simulink model "MMC_singlephase_test"  (Simulink 9.0)
settings: Solver=ode5  StartTime=0.0  StopTime=2  MaxStep=1e-4  RelTol=1e-3
libraries: powerlib x43
settings Model: Creator=lenovo  LastModifiedBy=lenovo
settings DataIOCC: SaveFormat=Dataset
settings OptimizationCC: LifeSpan=auto
settings DebuggingCC: UnderspecifiedInitializationDetection=Simplified  MergeDetectMultiDrivingBlocksExec=error  SFUnexpectedBacktrackingDiag=error  SFNoUnconditionalDefaultTransitionDiag=error  SFExecutionAtInitializationDiag=warning
settings HardwareCC: ProdBitPerPointer=64  ProdBitPerSizeT=64  ProdBitPerPtrDiffT=64  ProdLargestAtomicFloat=Float  ProdIntDivRoundTo=Zero  ProdEndianess=LittleEndian  ProdWordSize=64  ProdHWDeviceType=Intel->x86-64 (Windows64)
settings ModelReferenceCC: PropagateSignalLabelsOutOfModel=on
settings CodeAppCC: StateflowObjectComments=off
settings GRTTargetCC: TargetLangStandard=C99 (ISO)
settings ConfigComp: CovMetricSettings=dwe  CovHtmlReporting=off  CovSaveCumulativeToWorkspaceVar=off  CovSaveSingleToWorkspaceVar=off  CovExternalEMLEnable=on

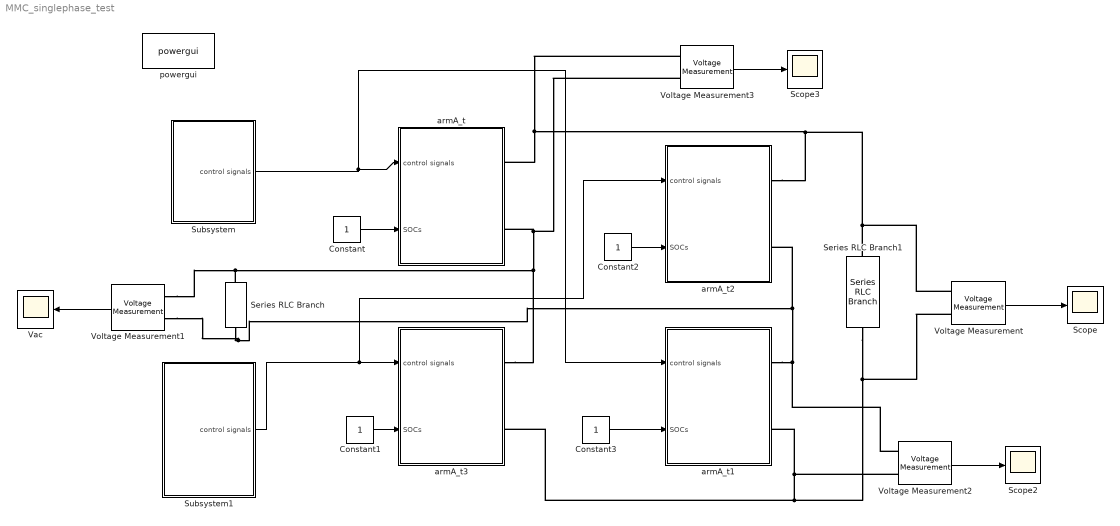
== system MMC_singlephase_test ==
  Constant{,1..3} (4 alike) : Constant
  Scope : Scope
  Scope2 : Scope
  Scope3 : Scope
  Series RLC Branch : powerlib/Elements/Series RLC Branch  LConnTagsString=__new0  RConnTagsString=__new0  BranchType=R  Resistance=1  Inductance=1e-3  SetiL0=off  InitialCurrent=0  Capacitance=1e-6  Setx0=off  InitialVoltage=0  Measurements=None
  Series RLC Branch1 : powerlib/Elements/Series RLC Branch  LConnTagsString=__new0  RConnTagsString=__new0  BranchType=R  Resistance=1  Inductance=1e-3  SetiL0=off  InitialCurrent=0  Capacitance=1e-6  Setx0=off  InitialVoltage=0  Measurements=None
  Subsystem : Subsystem
  Subsystem1 : Subsystem
  Vac : Scope
  Voltage Measurement{,1..3} (4 alike) : powerlib/Measurements/Voltage Measurement  PhasorSimulation=off  OutputType=Complex  PSBequivalent=0
  armA_t : Subsystem
  armA_t1 : Subsystem
  armA_t2 : Subsystem
  armA_t3 : Subsystem
  powergui : powerlib/powergui  Priority=1  SimulationMode=Discrete  SampleTime=50e-6  frequency=60  Iterations=50  frequencyindice=0  Pbase=100e6  ErrMax=1e-4  UnitsV=kV  UnitsW=MW  buscounter=0  FunctionMessages=off  echomessages=off  EnableUseOfTLC=off  CurrentSourceSwitches=off  DisableSnubberDevices=off  DisableRonSwitches=off  DisableVfSwitches=off  DisplayEquations=off  SolverType=Tustin/Backward Euler (TBE)  Interpol=off  ExternalGateDelay=off  methode=off  Ts=100  x0status=blocks  SPID=on  SwTol=0  HookPort=off  RestoreLinks=warning  ResistiveCurrentMeasurement=off  Frange=[0:2:500]  Ylog=off  Xlog=on  ShowGrid=off  save=off  variable=ZData  structure=0  ZoomFFT=off  StartTime=0.0  cycles=1  DisplayStyle=1  fundamental=60  FreqAxis=off  MaxFrequency=1000  frequencyindicesteady=1  RmsSteady=1  display=off
  wires:
  Voltage Measurement/1 -> Scope/1
  Subsystem/1(control signals) -> armA_t1/1(control signals), armA_t/1(control signals)
  Constant1/1 -> armA_t3/2(SOCs)
  Constant3/1 -> armA_t1/2(SOCs)
  Constant2/1 -> armA_t2/2(SOCs)
  Subsystem1/1(control signals) -> armA_t2/1(control signals), armA_t3/1(control signals)
  Voltage Measurement1/1 -> Vac/1
  Voltage Measurement2/1 -> Scope2/1
  Voltage Measurement3/1 -> Scope3/1
  Constant/1 -> armA_t/2(SOCs)
  connections:
  Series RLC Branch1/LConn1 -- Voltage Measurement/LConn1 -- armA_t/RConn1 -- Voltage Measurement3/LConn1 -- armA_t2/RConn1
  Series RLC Branch/LConn1 -- armA_t3/RConn1 -- armA_t/RConn2 -- Voltage Measurement3/LConn2 -- Voltage Measurement1/LConn1
  armA_t3/RConn2 -- Voltage Measurement/LConn2 -- Series RLC Branch1/RConn1 -- Voltage Measurement2/LConn2 -- armA_t1/RConn2
  Voltage Measurement1/LConn2 -- Series RLC Branch/RConn1 -- armA_t2/RConn2 -- armA_t1/RConn1 -- Voltage Measurement2/LConn1

== system MMC_singlephase_test/Subsystem ==
  Bus Creator : BusCreator  Inputs=3
  submodule1 : DiscretePulseGenerator  PulseType=Time based  Period=1  PulseWidth=75  PhaseDelay=0.125
  submodule2 : DiscretePulseGenerator  PulseType=Time based  Period=1  PulseWidth=50  PhaseDelay=0.25
  submodule3 : DiscretePulseGenerator  PulseType=Time based  Period=1  PulseWidth=25  PhaseDelay=0.375
  control signals : Outport
  wires:
  Bus Creator/1 -> control signals/1
  submodule1/1 -> Bus Creator/1
  submodule2/1 -> Bus Creator/2
  submodule3/1 -> Bus Creator/3

== system MMC_singlephase_test/Subsystem1 ==
  Bus Creator : BusCreator  Inputs=3
  Logical Operator : Logic  Operator=NOT  AllPortsSameDT=off  OutDataTypeStr=boolean
  Logical Operator1 : Logic  Operator=NOT  AllPortsSameDT=off  OutDataTypeStr=boolean
  Logical Operator2 : Logic  Operator=NOT  AllPortsSameDT=off  OutDataTypeStr=boolean
  submodule1 : DiscretePulseGenerator  PulseType=Time based  Period=1  PulseWidth=75  PhaseDelay=0.125
  submodule2 : DiscretePulseGenerator  PulseType=Time based  Period=1  PulseWidth=50  PhaseDelay=0.25
  submodule3 : DiscretePulseGenerator  PulseType=Time based  Period=1  PulseWidth=25  PhaseDelay=0.375
  control signals : Outport
  wires:
  Bus Creator/1 -> control signals/1
  submodule1/1 -> Logical Operator/1
  submodule2/1 -> Logical Operator1/1
  submodule3/1 -> Logical Operator2/1
  Logical Operator/1 -> Bus Creator/1
  Logical Operator1/1 -> Bus Creator/2
  Logical Operator2/1 -> Bus Creator/3

== system MMC_singlephase_test/armA_t ==
  control signals : Inport
  SOCs : Inport  Port=2
  Bus Selector : BusSelector  OutputSignals=signal1,signal2,signal3
  SubModule1 : Subsystem
  SubModule2 : Subsystem
  SubModule3 : Subsystem
  Conn1 : PMIOPort  Port=1  Side=Right
  Conn2 : PMIOPort  Port=2  Side=Right
  wires:
  control signals/1 -> Bus Selector/1
  SOCs/1 -> SubModule3/2(SOC), SubModule1/2(SOC), SubModule2/2(SOC)
  Bus Selector/2 -> SubModule2/1(control signal)  "<signal2>"
  Bus Selector/1 -> SubModule1/1(control signal)  "<signal1>"
  Bus Selector/3 -> SubModule3/1(control signal)  "<signal3>"
  connections:
  SubModule1/RConn2 -- SubModule2/RConn1
  SubModule1/RConn1 -- Conn1/RConn1
  Conn2/RConn1 -- SubModule3/RConn2
  SubModule2/RConn2 -- SubModule3/RConn1

== system MMC_singlephase_test/armA_t1 ==
  control signals : Inport
  SOCs : Inport  Port=2
  Bus Selector : BusSelector  OutputSignals=signal1,signal2,signal3
  SubModule1 : Subsystem
  SubModule2 : Subsystem
  SubModule3 : Subsystem
  Conn1 : PMIOPort  Port=1  Side=Right
  Conn2 : PMIOPort  Port=2  Side=Right
  wires:
  control signals/1 -> Bus Selector/1
  SOCs/1 -> SubModule3/2(SOC), SubModule1/2(SOC), SubModule2/2(SOC)
  Bus Selector/2 -> SubModule2/1(control signal)  "<signal2>"
  Bus Selector/1 -> SubModule1/1(control signal)  "<signal1>"
  Bus Selector/3 -> SubModule3/1(control signal)  "<signal3>"
  connections:
  SubModule1/RConn2 -- SubModule2/RConn1
  SubModule1/RConn1 -- Conn1/RConn1
  Conn2/RConn1 -- SubModule3/RConn2
  SubModule2/RConn2 -- SubModule3/RConn1

== system MMC_singlephase_test/armA_t2 ==
  control signals : Inport
  SOCs : Inport  Port=2
  Bus Selector : BusSelector  OutputSignals=signal1,signal2,signal3
  SubModule1 : Subsystem
  SubModule2 : Subsystem
  SubModule3 : Subsystem
  Conn1 : PMIOPort  Port=1  Side=Right
  Conn2 : PMIOPort  Port=2  Side=Right
  wires:
  control signals/1 -> Bus Selector/1
  SOCs/1 -> SubModule3/2(SOC), SubModule1/2(SOC), SubModule2/2(SOC)
  Bus Selector/2 -> SubModule2/1(control signal)  "<signal2>"
  Bus Selector/1 -> SubModule1/1(control signal)  "<signal1>"
  Bus Selector/3 -> SubModule3/1(control signal)  "<signal3>"
  connections:
  SubModule1/RConn2 -- SubModule2/RConn1
  SubModule1/RConn1 -- Conn1/RConn1
  Conn2/RConn1 -- SubModule3/RConn2
  SubModule2/RConn2 -- SubModule3/RConn1

== system MMC_singlephase_test/armA_t3 ==
  control signals : Inport
  SOCs : Inport  Port=2
  Bus Selector : BusSelector  OutputSignals=signal1,signal2,signal3
  SubModule1 : Subsystem
  SubModule2 : Subsystem
  SubModule3 : Subsystem
  Conn1 : PMIOPort  Port=1  Side=Right
  Conn2 : PMIOPort  Port=2  Side=Right
  wires:
  control signals/1 -> Bus Selector/1
  SOCs/1 -> SubModule3/2(SOC), SubModule1/2(SOC), SubModule2/2(SOC)
  Bus Selector/2 -> SubModule2/1(control signal)  "<signal2>"
  Bus Selector/1 -> SubModule1/1(control signal)  "<signal1>"
  Bus Selector/3 -> SubModule3/1(control signal)  "<signal3>"
  connections:
  SubModule1/RConn2 -- SubModule2/RConn1
  SubModule1/RConn1 -- Conn1/RConn1
  Conn2/RConn1 -- SubModule3/RConn2
  SubModule2/RConn2 -- SubModule3/RConn1

== system MMC_singlephase_test/armA_t/SubModule1 ==
  control signal : Inport
  SOC : Inport  Port=2
  MOSFET : Subsystem
  cell voltage : Subsystem
  P1 : PMIOPort  Tag=PMCPort  Port=1  Side=Right
  P2 : PMIOPort  Tag=PMCPort  Port=2  Side=Right
  wires:
  control signal/1 -> MOSFET/1(control signal)
  cell voltage/1(V) -> MOSFET/2(V)
  SOC/1 -> cell voltage/1(SOC)
  connections:
  P1/RConn1 -- MOSFET/RConn1
  P2/RConn1 -- MOSFET/RConn2

== system MMC_singlephase_test/armA_t/SubModule2 ==
  control signal : Inport
  SOC : Inport  Port=2
  MOSFET : Subsystem
  cell voltage : Subsystem
  P1 : PMIOPort  Tag=PMCPort  Port=1  Side=Right
  P2 : PMIOPort  Tag=PMCPort  Port=2  Side=Right
  wires:
  control signal/1 -> MOSFET/1(control signal)
  cell voltage/1(V) -> MOSFET/2(V)
  SOC/1 -> cell voltage/1(SOC)
  connections:
  P1/RConn1 -- MOSFET/RConn1
  P2/RConn1 -- MOSFET/RConn2

== system MMC_singlephase_test/armA_t/SubModule3 ==
  control signal : Inport
  SOC : Inport  Port=2
  MOSFET : Subsystem
  cell voltage : Subsystem
  P1 : PMIOPort  Tag=PMCPort  Port=1  Side=Right
  P2 : PMIOPort  Tag=PMCPort  Port=2  Side=Right
  wires:
  control signal/1 -> MOSFET/1(control signal)
  cell voltage/1(V) -> MOSFET/2(V)
  SOC/1 -> cell voltage/1(SOC)
  connections:
  P1/RConn1 -- MOSFET/RConn1
  P2/RConn1 -- MOSFET/RConn2

== system MMC_singlephase_test/armA_t1/SubModule1 ==
  control signal : Inport
  SOC : Inport  Port=2
  MOSFET : Subsystem
  cell voltage : Subsystem
  P1 : PMIOPort  Tag=PMCPort  Port=1  Side=Right
  P2 : PMIOPort  Tag=PMCPort  Port=2  Side=Right
  wires:
  control signal/1 -> MOSFET/1(control signal)
  cell voltage/1(V) -> MOSFET/2(V)
  SOC/1 -> cell voltage/1(SOC)
  connections:
  P1/RConn1 -- MOSFET/RConn1
  P2/RConn1 -- MOSFET/RConn2

== system MMC_singlephase_test/armA_t1/SubModule2 ==
  control signal : Inport
  SOC : Inport  Port=2
  MOSFET : Subsystem
  cell voltage : Subsystem
  P1 : PMIOPort  Tag=PMCPort  Port=1  Side=Right
  P2 : PMIOPort  Tag=PMCPort  Port=2  Side=Right
  wires:
  control signal/1 -> MOSFET/1(control signal)
  cell voltage/1(V) -> MOSFET/2(V)
  SOC/1 -> cell voltage/1(SOC)
  connections:
  P1/RConn1 -- MOSFET/RConn1
  P2/RConn1 -- MOSFET/RConn2

== system MMC_singlephase_test/armA_t1/SubModule3 ==
  control signal : Inport
  SOC : Inport  Port=2
  MOSFET : Subsystem
  cell voltage : Subsystem
  P1 : PMIOPort  Tag=PMCPort  Port=1  Side=Right
  P2 : PMIOPort  Tag=PMCPort  Port=2  Side=Right
  wires:
  control signal/1 -> MOSFET/1(control signal)
  cell voltage/1(V) -> MOSFET/2(V)
  SOC/1 -> cell voltage/1(SOC)
  connections:
  P1/RConn1 -- MOSFET/RConn1
  P2/RConn1 -- MOSFET/RConn2

== system MMC_singlephase_test/armA_t2/SubModule1 ==
  control signal : Inport
  SOC : Inport  Port=2
  MOSFET : Subsystem
  cell voltage : Subsystem
  P1 : PMIOPort  Tag=PMCPort  Port=1  Side=Right
  P2 : PMIOPort  Tag=PMCPort  Port=2  Side=Right
  wires:
  control signal/1 -> MOSFET/1(control signal)
  cell voltage/1(V) -> MOSFET/2(V)
  SOC/1 -> cell voltage/1(SOC)
  connections:
  P1/RConn1 -- MOSFET/RConn1
  P2/RConn1 -- MOSFET/RConn2

== system MMC_singlephase_test/armA_t2/SubModule2 ==
  control signal : Inport
  SOC : Inport  Port=2
  MOSFET : Subsystem
  cell voltage : Subsystem
  P1 : PMIOPort  Tag=PMCPort  Port=1  Side=Right
  P2 : PMIOPort  Tag=PMCPort  Port=2  Side=Right
  wires:
  control signal/1 -> MOSFET/1(control signal)
  cell voltage/1(V) -> MOSFET/2(V)
  SOC/1 -> cell voltage/1(SOC)
  connections:
  P1/RConn1 -- MOSFET/RConn1
  P2/RConn1 -- MOSFET/RConn2

== system MMC_singlephase_test/armA_t2/SubModule3 ==
  control signal : Inport
  SOC : Inport  Port=2
  MOSFET : Subsystem
  cell voltage : Subsystem
  P1 : PMIOPort  Tag=PMCPort  Port=1  Side=Right
  P2 : PMIOPort  Tag=PMCPort  Port=2  Side=Right
  wires:
  control signal/1 -> MOSFET/1(control signal)
  cell voltage/1(V) -> MOSFET/2(V)
  SOC/1 -> cell voltage/1(SOC)
  connections:
  P1/RConn1 -- MOSFET/RConn1
  P2/RConn1 -- MOSFET/RConn2

== system MMC_singlephase_test/armA_t3/SubModule1 ==
  control signal : Inport
  SOC : Inport  Port=2
  MOSFET : Subsystem
  cell voltage : Subsystem
  P1 : PMIOPort  Tag=PMCPort  Port=1  Side=Right
  P2 : PMIOPort  Tag=PMCPort  Port=2  Side=Right
  wires:
  control signal/1 -> MOSFET/1(control signal)
  cell voltage/1(V) -> MOSFET/2(V)
  SOC/1 -> cell voltage/1(SOC)
  connections:
  P1/RConn1 -- MOSFET/RConn1
  P2/RConn1 -- MOSFET/RConn2

== system MMC_singlephase_test/armA_t3/SubModule2 ==
  control signal : Inport
  SOC : Inport  Port=2
  MOSFET : Subsystem
  cell voltage : Subsystem
  P1 : PMIOPort  Tag=PMCPort  Port=1  Side=Right
  P2 : PMIOPort  Tag=PMCPort  Port=2  Side=Right
  wires:
  control signal/1 -> MOSFET/1(control signal)
  cell voltage/1(V) -> MOSFET/2(V)
  SOC/1 -> cell voltage/1(SOC)
  connections:
  P1/RConn1 -- MOSFET/RConn1
  P2/RConn1 -- MOSFET/RConn2

== system MMC_singlephase_test/armA_t3/SubModule3 ==
  control signal : Inport
  SOC : Inport  Port=2
  MOSFET : Subsystem
  cell voltage : Subsystem
  P1 : PMIOPort  Tag=PMCPort  Port=1  Side=Right
  P2 : PMIOPort  Tag=PMCPort  Port=2  Side=Right
  wires:
  control signal/1 -> MOSFET/1(control signal)
  cell voltage/1(V) -> MOSFET/2(V)
  SOC/1 -> cell voltage/1(SOC)
  connections:
  P1/RConn1 -- MOSFET/RConn1
  P2/RConn1 -- MOSFET/RConn2

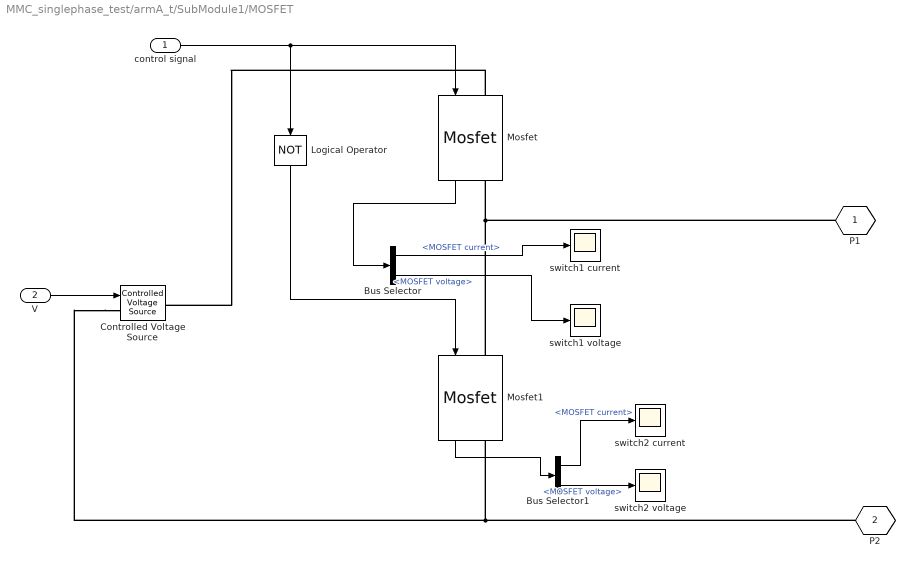
== system MMC_singlephase_test/armA_t/SubModule1/MOSFET ==
  control signal : Inport
  V : Inport  Port=2
  Bus Selector : BusSelector  OutputSignals=MOSFET current,MOSFET voltage
  Bus Selector1 : BusSelector  OutputSignals=MOSFET current,MOSFET voltage
  Controlled Voltage Source : powerlib/Electrical Sources/Controlled Voltage Source  Initialize=on  Source_Type=AC  Amplitude=0  Phase=0  Frequency=0  Measurements=None
  Logical Operator : Logic  Operator=NOT  AllPortsSameDT=off  OutDataTypeStr=boolean
  Mosfet : powerlib/Power Electronics/Mosfet  Ron=0.0005  Lon=0  Rd=0.01  Vfd=0  IC=0  Rs=1e5  Cs=inf  Measurements=on
  Mosfet1 : powerlib/Power Electronics/Mosfet  Ron=0.0005  Lon=0  Rd=0.01  Vfd=0  IC=0  Rs=1e5  Cs=inf  Measurements=on
  switch1 current : Scope
  switch1 voltage : Scope
  switch2 current : Scope
  switch2 voltage : Scope
  P1 : PMIOPort  Tag=PMCPort  Port=1  Side=Right
  P2 : PMIOPort  Tag=PMCPort  Port=2  Side=Right
  wires:
  control signal/1 -> Logical Operator/1, Mosfet/1
  Mosfet/1 -> Bus Selector/1
  V/1 -> Controlled Voltage Source/1
  Bus Selector/1 -> switch1 current/1  "<MOSFET current>"
  Bus Selector/2 -> switch1 voltage/1  "<MOSFET voltage>"
  Bus Selector1/1 -> switch2 current/1  "<MOSFET current>"
  Bus Selector1/2 -> switch2 voltage/1  "<MOSFET voltage>"
  Logical Operator/1 -> Mosfet1/1
  Mosfet1/1 -> Bus Selector1/1
  connections:
  Controlled Voltage Source/LConn1 -- Mosfet1/RConn1 -- P2/RConn1
  Mosfet1/LConn1 -- Mosfet/RConn1 -- P1/RConn1
  Mosfet/LConn1 -- Controlled Voltage Source/RConn1

== system MMC_singlephase_test/armA_t/SubModule1/cell voltage ==
  SOC : Inport
  Constant : Constant  Value=3
  Gain : Gain  Gain=1.2
  Sum : Sum  Inputs=|++
  V : Outport
  wires:
  Sum/1 -> V/1
  SOC/1 -> Gain/1
  Gain/1 -> Sum/2
  Constant/1 -> Sum/1

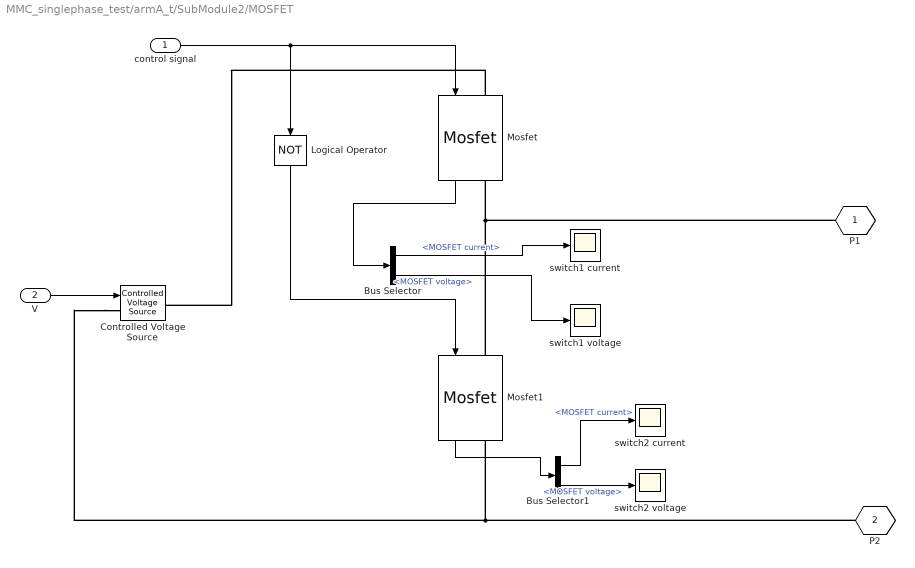
== system MMC_singlephase_test/armA_t/SubModule2/MOSFET ==
  control signal : Inport
  V : Inport  Port=2
  Bus Selector : BusSelector  OutputSignals=MOSFET current,MOSFET voltage
  Bus Selector1 : BusSelector  OutputSignals=MOSFET current,MOSFET voltage
  Controlled Voltage Source : powerlib/Electrical Sources/Controlled Voltage Source  Initialize=on  Source_Type=AC  Amplitude=0  Phase=0  Frequency=0  Measurements=None
  Logical Operator : Logic  Operator=NOT  AllPortsSameDT=off  OutDataTypeStr=boolean
  Mosfet : powerlib/Power Electronics/Mosfet  Ron=0.0005  Lon=0  Rd=0.01  Vfd=0  IC=0  Rs=1e5  Cs=inf  Measurements=on
  Mosfet1 : powerlib/Power Electronics/Mosfet  Ron=0.0005  Lon=0  Rd=0.01  Vfd=0  IC=0  Rs=1e5  Cs=inf  Measurements=on
  switch1 current : Scope
  switch1 voltage : Scope
  switch2 current : Scope
  switch2 voltage : Scope
  P1 : PMIOPort  Tag=PMCPort  Port=1  Side=Right
  P2 : PMIOPort  Tag=PMCPort  Port=2  Side=Right
  wires:
  control signal/1 -> Logical Operator/1, Mosfet/1
  Mosfet/1 -> Bus Selector/1
  V/1 -> Controlled Voltage Source/1
  Bus Selector/1 -> switch1 current/1  "<MOSFET current>"
  Bus Selector/2 -> switch1 voltage/1  "<MOSFET voltage>"
  Bus Selector1/1 -> switch2 current/1  "<MOSFET current>"
  Bus Selector1/2 -> switch2 voltage/1  "<MOSFET voltage>"
  Logical Operator/1 -> Mosfet1/1
  Mosfet1/1 -> Bus Selector1/1
  connections:
  Controlled Voltage Source/LConn1 -- Mosfet1/RConn1 -- P2/RConn1
  Mosfet1/LConn1 -- Mosfet/RConn1 -- P1/RConn1
  Mosfet/LConn1 -- Controlled Voltage Source/RConn1

== system MMC_singlephase_test/armA_t/SubModule2/cell voltage ==
  SOC : Inport
  Constant : Constant  Value=3
  Gain : Gain  Gain=1.2
  Sum : Sum  Inputs=|++
  V : Outport
  wires:
  Sum/1 -> V/1
  SOC/1 -> Gain/1
  Gain/1 -> Sum/2
  Constant/1 -> Sum/1

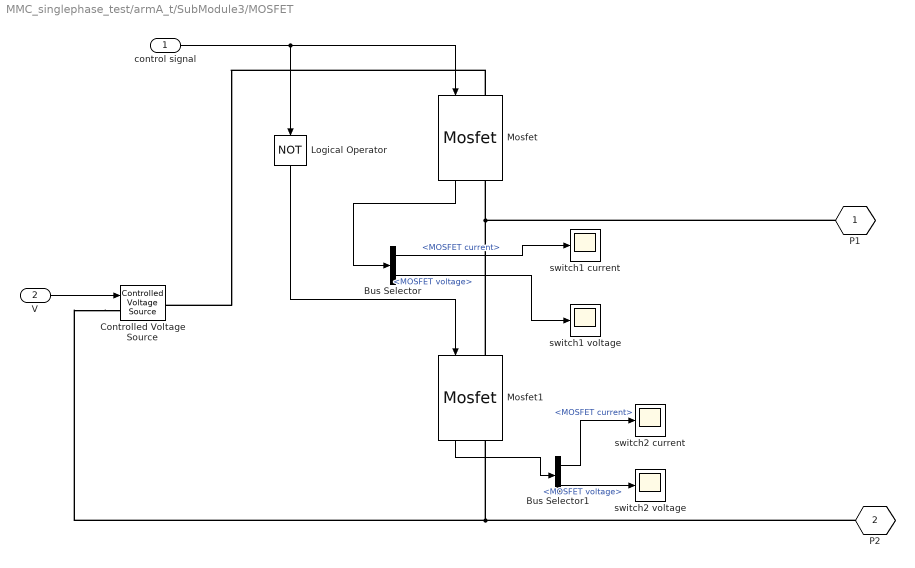
== system MMC_singlephase_test/armA_t/SubModule3/MOSFET ==
  control signal : Inport
  V : Inport  Port=2
  Bus Selector : BusSelector  OutputSignals=MOSFET current,MOSFET voltage
  Bus Selector1 : BusSelector  OutputSignals=MOSFET current,MOSFET voltage
  Controlled Voltage Source : powerlib/Electrical Sources/Controlled Voltage Source  Initialize=on  Source_Type=AC  Amplitude=0  Phase=0  Frequency=0  Measurements=None
  Logical Operator : Logic  Operator=NOT  AllPortsSameDT=off  OutDataTypeStr=boolean
  Mosfet : powerlib/Power Electronics/Mosfet  Ron=0.0005  Lon=0  Rd=0.01  Vfd=0  IC=0  Rs=1e5  Cs=inf  Measurements=on
  Mosfet1 : powerlib/Power Electronics/Mosfet  Ron=0.0005  Lon=0  Rd=0.01  Vfd=0  IC=0  Rs=1e5  Cs=inf  Measurements=on
  switch1 current : Scope
  switch1 voltage : Scope
  switch2 current : Scope
  switch2 voltage : Scope
  P1 : PMIOPort  Tag=PMCPort  Port=1  Side=Right
  P2 : PMIOPort  Tag=PMCPort  Port=2  Side=Right
  wires:
  control signal/1 -> Logical Operator/1, Mosfet/1
  Mosfet/1 -> Bus Selector/1
  V/1 -> Controlled Voltage Source/1
  Bus Selector/1 -> switch1 current/1  "<MOSFET current>"
  Bus Selector/2 -> switch1 voltage/1  "<MOSFET voltage>"
  Bus Selector1/1 -> switch2 current/1  "<MOSFET current>"
  Bus Selector1/2 -> switch2 voltage/1  "<MOSFET voltage>"
  Logical Operator/1 -> Mosfet1/1
  Mosfet1/1 -> Bus Selector1/1
  connections:
  Controlled Voltage Source/LConn1 -- Mosfet1/RConn1 -- P2/RConn1
  Mosfet1/LConn1 -- Mosfet/RConn1 -- P1/RConn1
  Mosfet/LConn1 -- Controlled Voltage Source/RConn1

== system MMC_singlephase_test/armA_t/SubModule3/cell voltage ==
  SOC : Inport
  Constant : Constant  Value=3
  Gain : Gain  Gain=1.2
  Sum : Sum  Inputs=|++
  V : Outport
  wires:
  Sum/1 -> V/1
  SOC/1 -> Gain/1
  Gain/1 -> Sum/2
  Constant/1 -> Sum/1

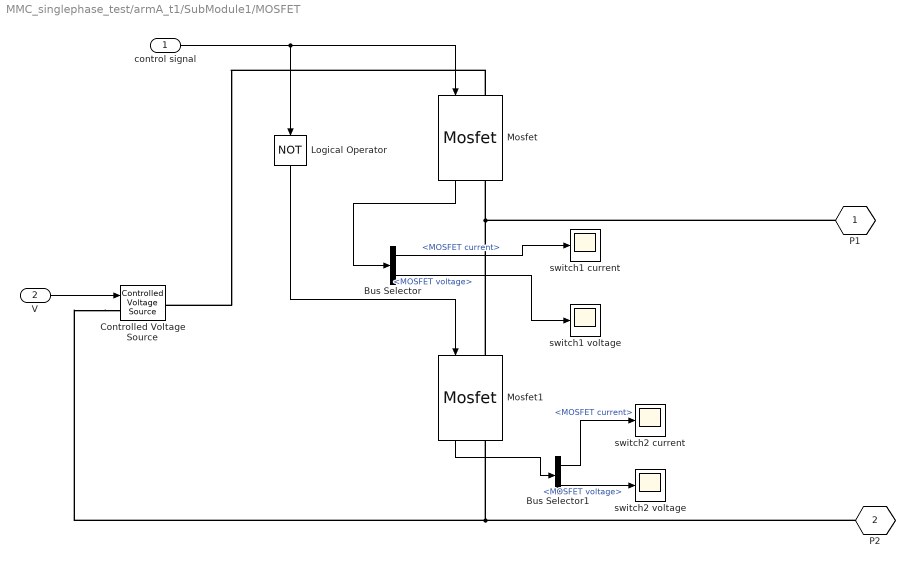
== system MMC_singlephase_test/armA_t1/SubModule1/MOSFET ==
  control signal : Inport
  V : Inport  Port=2
  Bus Selector : BusSelector  OutputSignals=MOSFET current,MOSFET voltage
  Bus Selector1 : BusSelector  OutputSignals=MOSFET current,MOSFET voltage
  Controlled Voltage Source : powerlib/Electrical Sources/Controlled Voltage Source  Initialize=on  Source_Type=AC  Amplitude=0  Phase=0  Frequency=0  Measurements=None
  Logical Operator : Logic  Operator=NOT  AllPortsSameDT=off  OutDataTypeStr=boolean
  Mosfet : powerlib/Power Electronics/Mosfet  Ron=0.0005  Lon=0  Rd=0.01  Vfd=0  IC=0  Rs=1e5  Cs=inf  Measurements=on
  Mosfet1 : powerlib/Power Electronics/Mosfet  Ron=0.0005  Lon=0  Rd=0.01  Vfd=0  IC=0  Rs=1e5  Cs=inf  Measurements=on
  switch1 current : Scope
  switch1 voltage : Scope
  switch2 current : Scope
  switch2 voltage : Scope
  P1 : PMIOPort  Tag=PMCPort  Port=1  Side=Right
  P2 : PMIOPort  Tag=PMCPort  Port=2  Side=Right
  wires:
  control signal/1 -> Logical Operator/1, Mosfet/1
  Mosfet/1 -> Bus Selector/1
  V/1 -> Controlled Voltage Source/1
  Bus Selector/1 -> switch1 current/1  "<MOSFET current>"
  Bus Selector/2 -> switch1 voltage/1  "<MOSFET voltage>"
  Bus Selector1/1 -> switch2 current/1  "<MOSFET current>"
  Bus Selector1/2 -> switch2 voltage/1  "<MOSFET voltage>"
  Logical Operator/1 -> Mosfet1/1
  Mosfet1/1 -> Bus Selector1/1
  connections:
  Controlled Voltage Source/LConn1 -- Mosfet1/RConn1 -- P2/RConn1
  Mosfet1/LConn1 -- Mosfet/RConn1 -- P1/RConn1
  Mosfet/LConn1 -- Controlled Voltage Source/RConn1

== system MMC_singlephase_test/armA_t1/SubModule1/cell voltage ==
  SOC : Inport
  Constant : Constant  Value=3
  Gain : Gain  Gain=1.2
  Sum : Sum  Inputs=|++
  V : Outport
  wires:
  Sum/1 -> V/1
  SOC/1 -> Gain/1
  Gain/1 -> Sum/2
  Constant/1 -> Sum/1

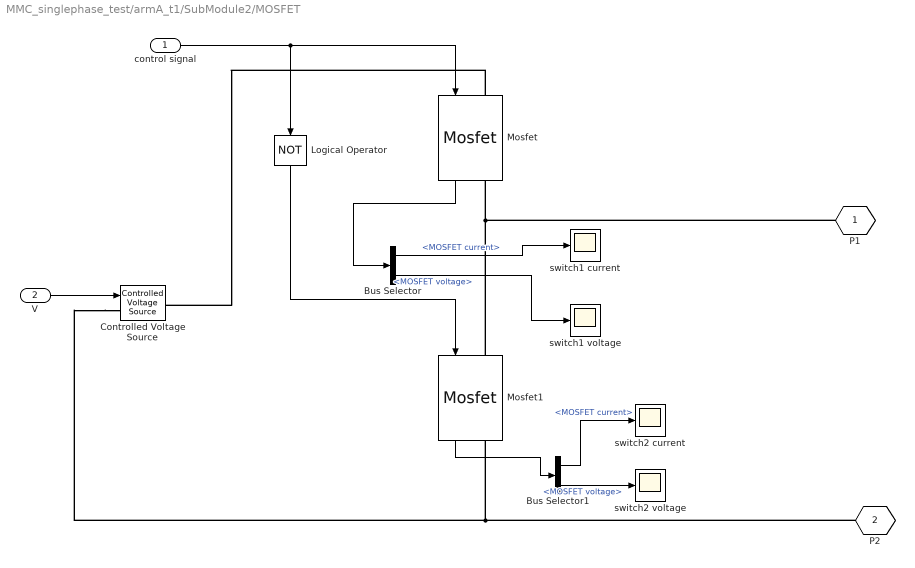
== system MMC_singlephase_test/armA_t1/SubModule2/MOSFET ==
  control signal : Inport
  V : Inport  Port=2
  Bus Selector : BusSelector  OutputSignals=MOSFET current,MOSFET voltage
  Bus Selector1 : BusSelector  OutputSignals=MOSFET current,MOSFET voltage
  Controlled Voltage Source : powerlib/Electrical Sources/Controlled Voltage Source  Initialize=on  Source_Type=AC  Amplitude=0  Phase=0  Frequency=0  Measurements=None
  Logical Operator : Logic  Operator=NOT  AllPortsSameDT=off  OutDataTypeStr=boolean
  Mosfet : powerlib/Power Electronics/Mosfet  Ron=0.0005  Lon=0  Rd=0.01  Vfd=0  IC=0  Rs=1e5  Cs=inf  Measurements=on
  Mosfet1 : powerlib/Power Electronics/Mosfet  Ron=0.0005  Lon=0  Rd=0.01  Vfd=0  IC=0  Rs=1e5  Cs=inf  Measurements=on
  switch1 current : Scope
  switch1 voltage : Scope
  switch2 current : Scope
  switch2 voltage : Scope
  P1 : PMIOPort  Tag=PMCPort  Port=1  Side=Right
  P2 : PMIOPort  Tag=PMCPort  Port=2  Side=Right
  wires:
  control signal/1 -> Logical Operator/1, Mosfet/1
  Mosfet/1 -> Bus Selector/1
  V/1 -> Controlled Voltage Source/1
  Bus Selector/1 -> switch1 current/1  "<MOSFET current>"
  Bus Selector/2 -> switch1 voltage/1  "<MOSFET voltage>"
  Bus Selector1/1 -> switch2 current/1  "<MOSFET current>"
  Bus Selector1/2 -> switch2 voltage/1  "<MOSFET voltage>"
  Logical Operator/1 -> Mosfet1/1
  Mosfet1/1 -> Bus Selector1/1
  connections:
  Controlled Voltage Source/LConn1 -- Mosfet1/RConn1 -- P2/RConn1
  Mosfet1/LConn1 -- Mosfet/RConn1 -- P1/RConn1
  Mosfet/LConn1 -- Controlled Voltage Source/RConn1

== system MMC_singlephase_test/armA_t1/SubModule2/cell voltage ==
  SOC : Inport
  Constant : Constant  Value=3
  Gain : Gain  Gain=1.2
  Sum : Sum  Inputs=|++
  V : Outport
  wires:
  Sum/1 -> V/1
  SOC/1 -> Gain/1
  Gain/1 -> Sum/2
  Constant/1 -> Sum/1

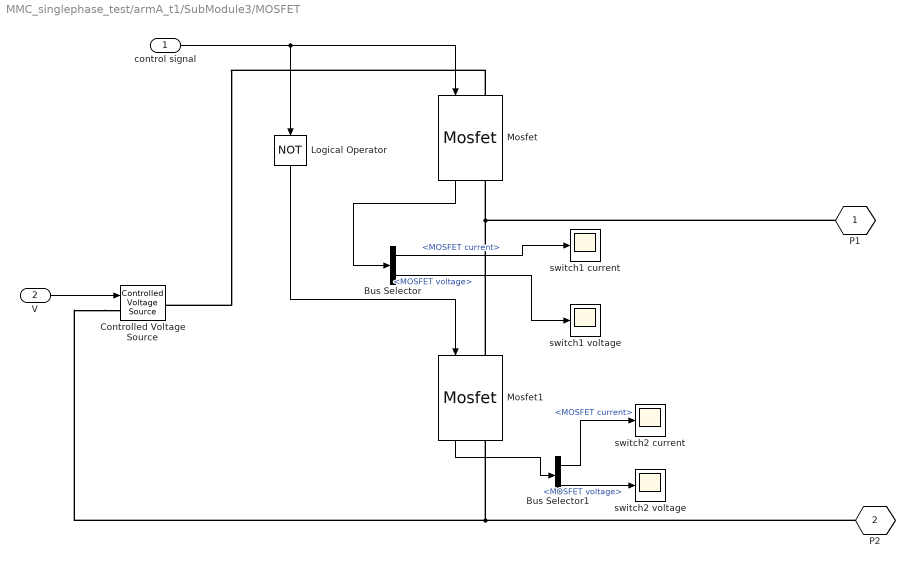
== system MMC_singlephase_test/armA_t1/SubModule3/MOSFET ==
  control signal : Inport
  V : Inport  Port=2
  Bus Selector : BusSelector  OutputSignals=MOSFET current,MOSFET voltage
  Bus Selector1 : BusSelector  OutputSignals=MOSFET current,MOSFET voltage
  Controlled Voltage Source : powerlib/Electrical Sources/Controlled Voltage Source  Initialize=on  Source_Type=AC  Amplitude=0  Phase=0  Frequency=0  Measurements=None
  Logical Operator : Logic  Operator=NOT  AllPortsSameDT=off  OutDataTypeStr=boolean
  Mosfet : powerlib/Power Electronics/Mosfet  Ron=0.0005  Lon=0  Rd=0.01  Vfd=0  IC=0  Rs=1e5  Cs=inf  Measurements=on
  Mosfet1 : powerlib/Power Electronics/Mosfet  Ron=0.0005  Lon=0  Rd=0.01  Vfd=0  IC=0  Rs=1e5  Cs=inf  Measurements=on
  switch1 current : Scope
  switch1 voltage : Scope
  switch2 current : Scope
  switch2 voltage : Scope
  P1 : PMIOPort  Tag=PMCPort  Port=1  Side=Right
  P2 : PMIOPort  Tag=PMCPort  Port=2  Side=Right
  wires:
  control signal/1 -> Logical Operator/1, Mosfet/1
  Mosfet/1 -> Bus Selector/1
  V/1 -> Controlled Voltage Source/1
  Bus Selector/1 -> switch1 current/1  "<MOSFET current>"
  Bus Selector/2 -> switch1 voltage/1  "<MOSFET voltage>"
  Bus Selector1/1 -> switch2 current/1  "<MOSFET current>"
  Bus Selector1/2 -> switch2 voltage/1  "<MOSFET voltage>"
  Logical Operator/1 -> Mosfet1/1
  Mosfet1/1 -> Bus Selector1/1
  connections:
  Controlled Voltage Source/LConn1 -- Mosfet1/RConn1 -- P2/RConn1
  Mosfet1/LConn1 -- Mosfet/RConn1 -- P1/RConn1
  Mosfet/LConn1 -- Controlled Voltage Source/RConn1

== system MMC_singlephase_test/armA_t1/SubModule3/cell voltage ==
  SOC : Inport
  Constant : Constant  Value=3
  Gain : Gain  Gain=1.2
  Sum : Sum  Inputs=|++
  V : Outport
  wires:
  Sum/1 -> V/1
  SOC/1 -> Gain/1
  Gain/1 -> Sum/2
  Constant/1 -> Sum/1

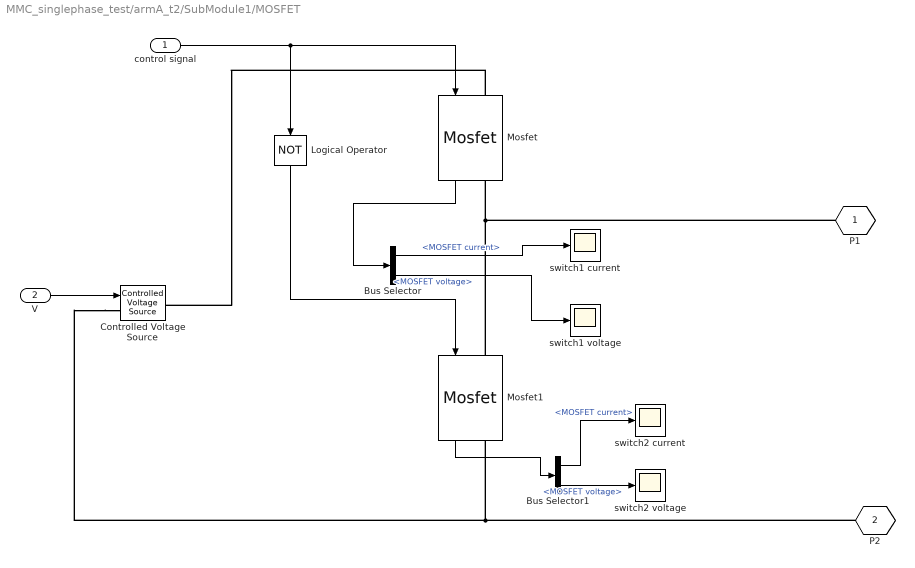
== system MMC_singlephase_test/armA_t2/SubModule1/MOSFET ==
  control signal : Inport
  V : Inport  Port=2
  Bus Selector : BusSelector  OutputSignals=MOSFET current,MOSFET voltage
  Bus Selector1 : BusSelector  OutputSignals=MOSFET current,MOSFET voltage
  Controlled Voltage Source : powerlib/Electrical Sources/Controlled Voltage Source  Initialize=on  Source_Type=AC  Amplitude=0  Phase=0  Frequency=0  Measurements=None
  Logical Operator : Logic  Operator=NOT  AllPortsSameDT=off  OutDataTypeStr=boolean
  Mosfet : powerlib/Power Electronics/Mosfet  Ron=0.0005  Lon=0  Rd=0.01  Vfd=0  IC=0  Rs=1e5  Cs=inf  Measurements=on
  Mosfet1 : powerlib/Power Electronics/Mosfet  Ron=0.0005  Lon=0  Rd=0.01  Vfd=0  IC=0  Rs=1e5  Cs=inf  Measurements=on
  switch1 current : Scope
  switch1 voltage : Scope
  switch2 current : Scope
  switch2 voltage : Scope
  P1 : PMIOPort  Tag=PMCPort  Port=1  Side=Right
  P2 : PMIOPort  Tag=PMCPort  Port=2  Side=Right
  wires:
  control signal/1 -> Logical Operator/1, Mosfet/1
  Mosfet/1 -> Bus Selector/1
  V/1 -> Controlled Voltage Source/1
  Bus Selector/1 -> switch1 current/1  "<MOSFET current>"
  Bus Selector/2 -> switch1 voltage/1  "<MOSFET voltage>"
  Bus Selector1/1 -> switch2 current/1  "<MOSFET current>"
  Bus Selector1/2 -> switch2 voltage/1  "<MOSFET voltage>"
  Logical Operator/1 -> Mosfet1/1
  Mosfet1/1 -> Bus Selector1/1
  connections:
  Controlled Voltage Source/LConn1 -- Mosfet1/RConn1 -- P2/RConn1
  Mosfet1/LConn1 -- Mosfet/RConn1 -- P1/RConn1
  Mosfet/LConn1 -- Controlled Voltage Source/RConn1

== system MMC_singlephase_test/armA_t2/SubModule1/cell voltage ==
  SOC : Inport
  Constant : Constant  Value=3
  Gain : Gain  Gain=1.2
  Sum : Sum  Inputs=|++
  V : Outport
  wires:
  Sum/1 -> V/1
  SOC/1 -> Gain/1
  Gain/1 -> Sum/2
  Constant/1 -> Sum/1

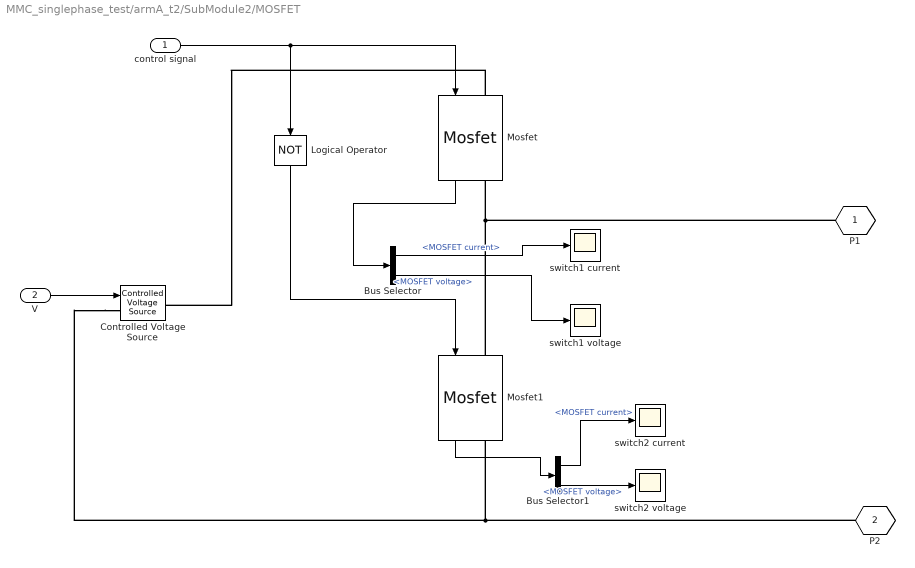
== system MMC_singlephase_test/armA_t2/SubModule2/MOSFET ==
  control signal : Inport
  V : Inport  Port=2
  Bus Selector : BusSelector  OutputSignals=MOSFET current,MOSFET voltage
  Bus Selector1 : BusSelector  OutputSignals=MOSFET current,MOSFET voltage
  Controlled Voltage Source : powerlib/Electrical Sources/Controlled Voltage Source  Initialize=on  Source_Type=AC  Amplitude=0  Phase=0  Frequency=0  Measurements=None
  Logical Operator : Logic  Operator=NOT  AllPortsSameDT=off  OutDataTypeStr=boolean
  Mosfet : powerlib/Power Electronics/Mosfet  Ron=0.0005  Lon=0  Rd=0.01  Vfd=0  IC=0  Rs=1e5  Cs=inf  Measurements=on
  Mosfet1 : powerlib/Power Electronics/Mosfet  Ron=0.0005  Lon=0  Rd=0.01  Vfd=0  IC=0  Rs=1e5  Cs=inf  Measurements=on
  switch1 current : Scope
  switch1 voltage : Scope
  switch2 current : Scope
  switch2 voltage : Scope
  P1 : PMIOPort  Tag=PMCPort  Port=1  Side=Right
  P2 : PMIOPort  Tag=PMCPort  Port=2  Side=Right
  wires:
  control signal/1 -> Logical Operator/1, Mosfet/1
  Mosfet/1 -> Bus Selector/1
  V/1 -> Controlled Voltage Source/1
  Bus Selector/1 -> switch1 current/1  "<MOSFET current>"
  Bus Selector/2 -> switch1 voltage/1  "<MOSFET voltage>"
  Bus Selector1/1 -> switch2 current/1  "<MOSFET current>"
  Bus Selector1/2 -> switch2 voltage/1  "<MOSFET voltage>"
  Logical Operator/1 -> Mosfet1/1
  Mosfet1/1 -> Bus Selector1/1
  connections:
  Controlled Voltage Source/LConn1 -- Mosfet1/RConn1 -- P2/RConn1
  Mosfet1/LConn1 -- Mosfet/RConn1 -- P1/RConn1
  Mosfet/LConn1 -- Controlled Voltage Source/RConn1

== system MMC_singlephase_test/armA_t2/SubModule2/cell voltage ==
  SOC : Inport
  Constant : Constant  Value=3
  Gain : Gain  Gain=1.2
  Sum : Sum  Inputs=|++
  V : Outport
  wires:
  Sum/1 -> V/1
  SOC/1 -> Gain/1
  Gain/1 -> Sum/2
  Constant/1 -> Sum/1

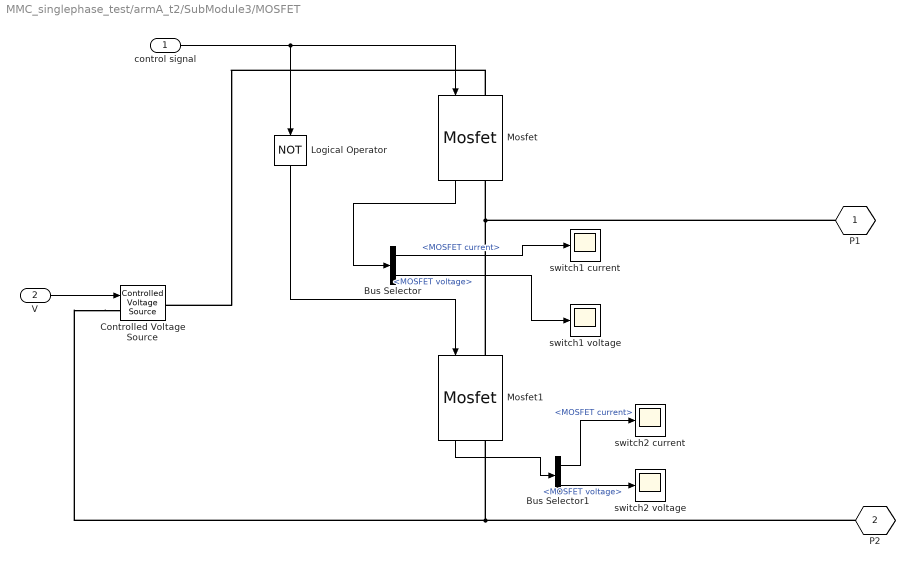
== system MMC_singlephase_test/armA_t2/SubModule3/MOSFET ==
  control signal : Inport
  V : Inport  Port=2
  Bus Selector : BusSelector  OutputSignals=MOSFET current,MOSFET voltage
  Bus Selector1 : BusSelector  OutputSignals=MOSFET current,MOSFET voltage
  Controlled Voltage Source : powerlib/Electrical Sources/Controlled Voltage Source  Initialize=on  Source_Type=AC  Amplitude=0  Phase=0  Frequency=0  Measurements=None
  Logical Operator : Logic  Operator=NOT  AllPortsSameDT=off  OutDataTypeStr=boolean
  Mosfet : powerlib/Power Electronics/Mosfet  Ron=0.0005  Lon=0  Rd=0.01  Vfd=0  IC=0  Rs=1e5  Cs=inf  Measurements=on
  Mosfet1 : powerlib/Power Electronics/Mosfet  Ron=0.0005  Lon=0  Rd=0.01  Vfd=0  IC=0  Rs=1e5  Cs=inf  Measurements=on
  switch1 current : Scope
  switch1 voltage : Scope
  switch2 current : Scope
  switch2 voltage : Scope
  P1 : PMIOPort  Tag=PMCPort  Port=1  Side=Right
  P2 : PMIOPort  Tag=PMCPort  Port=2  Side=Right
  wires:
  control signal/1 -> Logical Operator/1, Mosfet/1
  Mosfet/1 -> Bus Selector/1
  V/1 -> Controlled Voltage Source/1
  Bus Selector/1 -> switch1 current/1  "<MOSFET current>"
  Bus Selector/2 -> switch1 voltage/1  "<MOSFET voltage>"
  Bus Selector1/1 -> switch2 current/1  "<MOSFET current>"
  Bus Selector1/2 -> switch2 voltage/1  "<MOSFET voltage>"
  Logical Operator/1 -> Mosfet1/1
  Mosfet1/1 -> Bus Selector1/1
  connections:
  Controlled Voltage Source/LConn1 -- Mosfet1/RConn1 -- P2/RConn1
  Mosfet1/LConn1 -- Mosfet/RConn1 -- P1/RConn1
  Mosfet/LConn1 -- Controlled Voltage Source/RConn1

== system MMC_singlephase_test/armA_t2/SubModule3/cell voltage ==
  SOC : Inport
  Constant : Constant  Value=3
  Gain : Gain  Gain=1.2
  Sum : Sum  Inputs=|++
  V : Outport
  wires:
  Sum/1 -> V/1
  SOC/1 -> Gain/1
  Gain/1 -> Sum/2
  Constant/1 -> Sum/1

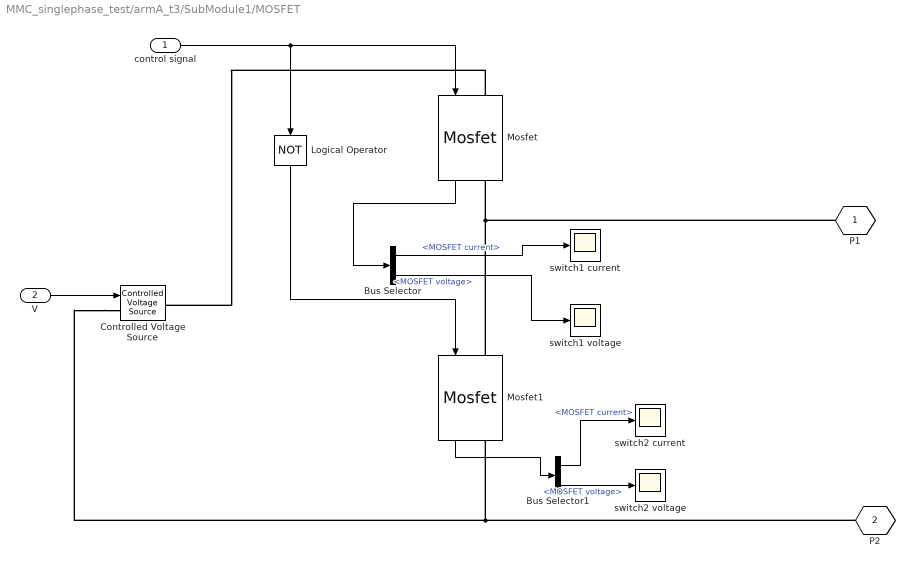
== system MMC_singlephase_test/armA_t3/SubModule1/MOSFET ==
  control signal : Inport
  V : Inport  Port=2
  Bus Selector : BusSelector  OutputSignals=MOSFET current,MOSFET voltage
  Bus Selector1 : BusSelector  OutputSignals=MOSFET current,MOSFET voltage
  Controlled Voltage Source : powerlib/Electrical Sources/Controlled Voltage Source  Initialize=on  Source_Type=AC  Amplitude=0  Phase=0  Frequency=0  Measurements=None
  Logical Operator : Logic  Operator=NOT  AllPortsSameDT=off  OutDataTypeStr=boolean
  Mosfet : powerlib/Power Electronics/Mosfet  Ron=0.0005  Lon=0  Rd=0.01  Vfd=0  IC=0  Rs=1e5  Cs=inf  Measurements=on
  Mosfet1 : powerlib/Power Electronics/Mosfet  Ron=0.0005  Lon=0  Rd=0.01  Vfd=0  IC=0  Rs=1e5  Cs=inf  Measurements=on
  switch1 current : Scope
  switch1 voltage : Scope
  switch2 current : Scope
  switch2 voltage : Scope
  P1 : PMIOPort  Tag=PMCPort  Port=1  Side=Right
  P2 : PMIOPort  Tag=PMCPort  Port=2  Side=Right
  wires:
  control signal/1 -> Logical Operator/1, Mosfet/1
  Mosfet/1 -> Bus Selector/1
  V/1 -> Controlled Voltage Source/1
  Bus Selector/1 -> switch1 current/1  "<MOSFET current>"
  Bus Selector/2 -> switch1 voltage/1  "<MOSFET voltage>"
  Bus Selector1/1 -> switch2 current/1  "<MOSFET current>"
  Bus Selector1/2 -> switch2 voltage/1  "<MOSFET voltage>"
  Logical Operator/1 -> Mosfet1/1
  Mosfet1/1 -> Bus Selector1/1
  connections:
  Controlled Voltage Source/LConn1 -- Mosfet1/RConn1 -- P2/RConn1
  Mosfet1/LConn1 -- Mosfet/RConn1 -- P1/RConn1
  Mosfet/LConn1 -- Controlled Voltage Source/RConn1

== system MMC_singlephase_test/armA_t3/SubModule1/cell voltage ==
  SOC : Inport
  Constant : Constant  Value=3
  Gain : Gain  Gain=1.2
  Sum : Sum  Inputs=|++
  V : Outport
  wires:
  Sum/1 -> V/1
  SOC/1 -> Gain/1
  Gain/1 -> Sum/2
  Constant/1 -> Sum/1

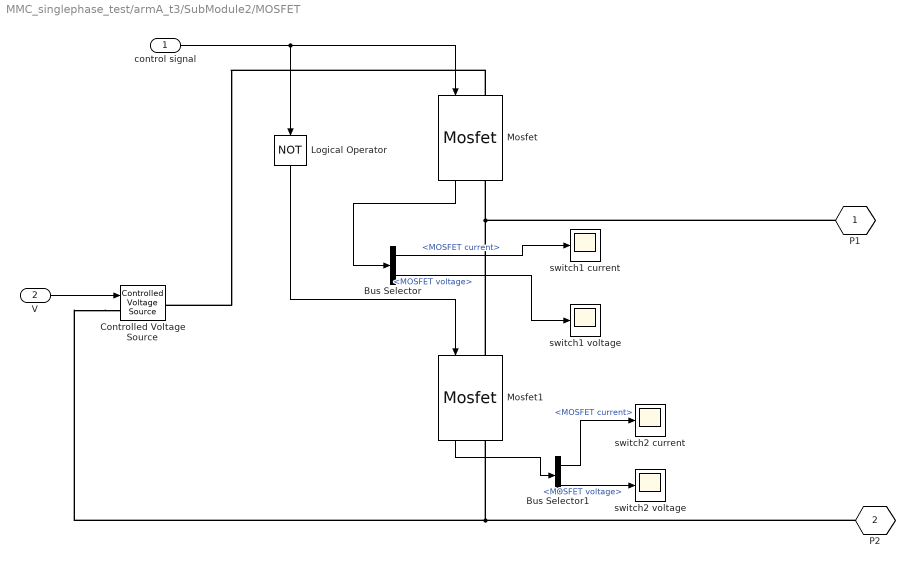
== system MMC_singlephase_test/armA_t3/SubModule2/MOSFET ==
  control signal : Inport
  V : Inport  Port=2
  Bus Selector : BusSelector  OutputSignals=MOSFET current,MOSFET voltage
  Bus Selector1 : BusSelector  OutputSignals=MOSFET current,MOSFET voltage
  Controlled Voltage Source : powerlib/Electrical Sources/Controlled Voltage Source  Initialize=on  Source_Type=AC  Amplitude=0  Phase=0  Frequency=0  Measurements=None
  Logical Operator : Logic  Operator=NOT  AllPortsSameDT=off  OutDataTypeStr=boolean
  Mosfet : powerlib/Power Electronics/Mosfet  Ron=0.0005  Lon=0  Rd=0.01  Vfd=0  IC=0  Rs=1e5  Cs=inf  Measurements=on
  Mosfet1 : powerlib/Power Electronics/Mosfet  Ron=0.0005  Lon=0  Rd=0.01  Vfd=0  IC=0  Rs=1e5  Cs=inf  Measurements=on
  switch1 current : Scope
  switch1 voltage : Scope
  switch2 current : Scope
  switch2 voltage : Scope
  P1 : PMIOPort  Tag=PMCPort  Port=1  Side=Right
  P2 : PMIOPort  Tag=PMCPort  Port=2  Side=Right
  wires:
  control signal/1 -> Logical Operator/1, Mosfet/1
  Mosfet/1 -> Bus Selector/1
  V/1 -> Controlled Voltage Source/1
  Bus Selector/1 -> switch1 current/1  "<MOSFET current>"
  Bus Selector/2 -> switch1 voltage/1  "<MOSFET voltage>"
  Bus Selector1/1 -> switch2 current/1  "<MOSFET current>"
  Bus Selector1/2 -> switch2 voltage/1  "<MOSFET voltage>"
  Logical Operator/1 -> Mosfet1/1
  Mosfet1/1 -> Bus Selector1/1
  connections:
  Controlled Voltage Source/LConn1 -- Mosfet1/RConn1 -- P2/RConn1
  Mosfet1/LConn1 -- Mosfet/RConn1 -- P1/RConn1
  Mosfet/LConn1 -- Controlled Voltage Source/RConn1

== system MMC_singlephase_test/armA_t3/SubModule2/cell voltage ==
  SOC : Inport
  Constant : Constant  Value=3
  Gain : Gain  Gain=1.2
  Sum : Sum  Inputs=|++
  V : Outport
  wires:
  Sum/1 -> V/1
  SOC/1 -> Gain/1
  Gain/1 -> Sum/2
  Constant/1 -> Sum/1

== system MMC_singlephase_test/armA_t3/SubModule3/MOSFET ==
  control signal : Inport
  V : Inport  Port=2
  Bus Selector : BusSelector  OutputSignals=MOSFET current,MOSFET voltage
  Bus Selector1 : BusSelector  OutputSignals=MOSFET current,MOSFET voltage
  Controlled Voltage Source : powerlib/Electrical Sources/Controlled Voltage Source  Initialize=on  Source_Type=AC  Amplitude=0  Phase=0  Frequency=0  Measurements=None
  Logical Operator : Logic  Operator=NOT  AllPortsSameDT=off  OutDataTypeStr=boolean
  Mosfet : powerlib/Power Electronics/Mosfet  Ron=0.0005  Lon=0  Rd=0.01  Vfd=0  IC=0  Rs=1e5  Cs=inf  Measurements=on
  Mosfet1 : powerlib/Power Electronics/Mosfet  Ron=0.0005  Lon=0  Rd=0.01  Vfd=0  IC=0  Rs=1e5  Cs=inf  Measurements=on
  switch1 current : Scope
  switch1 voltage : Scope
  switch2 current : Scope
  switch2 voltage : Scope
  P1 : PMIOPort  Tag=PMCPort  Port=1  Side=Right
  P2 : PMIOPort  Tag=PMCPort  Port=2  Side=Right
  wires:
  control signal/1 -> Logical Operator/1, Mosfet/1
  Mosfet/1 -> Bus Selector/1
  V/1 -> Controlled Voltage Source/1
  Bus Selector/1 -> switch1 current/1  "<MOSFET current>"
  Bus Selector/2 -> switch1 voltage/1  "<MOSFET voltage>"
  Bus Selector1/1 -> switch2 current/1  "<MOSFET current>"
  Bus Selector1/2 -> switch2 voltage/1  "<MOSFET voltage>"
  Logical Operator/1 -> Mosfet1/1
  Mosfet1/1 -> Bus Selector1/1
  connections:
  Controlled Voltage Source/LConn1 -- Mosfet1/RConn1 -- P2/RConn1
  Mosfet1/LConn1 -- Mosfet/RConn1 -- P1/RConn1
  Mosfet/LConn1 -- Controlled Voltage Source/RConn1

== system MMC_singlephase_test/armA_t3/SubModule3/cell voltage ==
  SOC : Inport
  Constant : Constant  Value=3
  Gain : Gain  Gain=1.2
  Sum : Sum  Inputs=|++
  V : Outport
  wires:
  Sum/1 -> V/1
  SOC/1 -> Gain/1
  Gain/1 -> Sum/2
  Constant/1 -> Sum/1
